simulink model "IMP_LQR_2018_Dist_Mult"  (R2018a)
settings: Solver=ode1  StartTime=0.0  StopTime=20  FixedStep=0.002  RelTol=1e-3  EnableMultiTasking=on
values from neighbouring files (symbols this model uses):
  A = [0 0 1 0 ... (first row only)    [IMP_LQR_Design_2.m]    (also in IMP_LQR_Design_C.m; IMP_LQR_Design_SepPrinc.m; IMP_LQR_Design_Seperation.m; IMP_LQR_Design_Seperation_Compare.m)
  A_aug = [A B*Cref; zeros(4,4) Aref]    [IMP_LQR_Design_2.m]    (also in IMP_LQR_Design_C.m; IMP_LQR_Design_SepPrinc.m; IMP_LQR_Design_Seperation.m; IMP_LQR_Design_Seperation_Compare.m)
  B = [0 0; 0 0; Kpp/Jp Kpy/Jp; Kyp/Jy Kyy/Jy]    [IMP_LQR_Design_2.m]    (also in IMP_LQR_Design_C.m; IMP_LQR_Design_SepPrinc.m; IMP_LQR_Design_Seperation.m; IMP_LQR_Design_Seperation_Compare.m)
  B_aug = [B; zeros(4,2)]    [IMP_LQR_Design_2.m]    (also in IMP_LQR_Design_C.m; IMP_LQR_Design_SepPrinc.m; IMP_LQR_Design_Seperation.m; IMP_LQR_Design_Seperation_Compare.m)
  C = [1 0 0 0; 0 1 0 0]    [IMP_LQR_Design_2.m]    (also in IMP_LQR_Design_C.m; IMP_LQR_Design_SepPrinc.m = [0 0 1 0; 0 1 0 0]; IMP_LQR_Design_Seperation.m; IMP_LQR_Design_Seperation_Compare.m = [0 1 0 0; 0 1 0 0])
  C_aug = [C zeros(2,4)]    [IMP_LQR_Design_2.m]    (also in IMP_LQR_Design_C.m; IMP_LQR_Design_SepPrinc.m; IMP_LQR_Design_Seperation.m; IMP_LQR_Design_Seperation_Compare.m)
  J = [J;J]    [IMP_LQR_Design_2.m]    (also in IMP_LQR_Design_C.m; IMP_LQR_Design_Seperation.m = J'; IMP_LQR_Design_Seperation_Compare.m = J'; design_C.m = place(A',C', polesj)')
  K = [K Cref]    [IMP_LQR_Design_2.m]    (also in IMP_LQR_Design_C.m; IMP_LQR_Design_SepPrinc.m; IMP_LQR_Design_Seperation.m; IMP_LQR_Design_Seperation_Compare.m)
  N = K(1:2,1:2)    [IMP_LQR_Design_2.m]    (also in IMP_LQR_Design_C.m; IMP_LQR_Design_SepPrinc.m; IMP_LQR_Design_Seperation.m; IMP_LQR_Design_Seperation_Compare.m)
  wo = 30    [IMP_LQR_Design_Seperation.m]    (also in IMP_LQR_Design_Seperation_Compare.m)
libraries: simulink x4, simulink_extras x4, dspsrcs4 x1
settings Model: ExtModeTrigDuration=5000  Creator=MLevis  LastModifiedBy=jakelangton
settings SolverCC: PositivePriorityOrder=on
settings DataIOCC: LimitDataPoints=on  SaveFormat=Array
settings OptimizationCC: LifeSpan=inf
settings DebuggingCC: SolverPrmCheckMsg=warning  SFUnexpectedBacktrackingDiag=warning  SFNoUnconditionalDefaultTransitionDiag=warning  SFExecutionAtInitializationDiag=none
settings HardwareCC: ProdBitPerPointer=32  ProdBitPerSizeT=32  ProdBitPerPtrDiffT=32  ProdLargestAtomicFloat=None  ProdIntDivRoundTo=Undefined  ProdEndianess=Unspecified  ProdWordSize=32  ProdHWDeviceType=32-bit Generic
settings ModelReferenceCC: PropagateSignalLabelsOutOfModel=off
settings RTWCC: SystemTargetFile=quarc_win64.tlc  TemplateMakefile=quarc_default_tmf  Description=QUARC Win64 Target
settings CodeAppCC: StateflowObjectComments=on
settings STFCustomTargetCC: TargetPreCompLibLocation=C:\PROGRA~3\QUARC\lib\2014a\win64\release  ConcurrentExecutionCompliant=on  GeneratePreprocessorConditionals=Disable all  SystemTargetFile=quarc_win64.tlc
settings GRTTargetCC: TargetPreCompLibLocation=C:\PROGRA~3\QUARC\lib\2014a\win64\release  TargetLangStandard=C89/C90 (ANSI)  ParMdlRefBuildCompliant=off  CompOptLevelCompliant=off  GeneratePreprocessorConditionals=Disable all  CombineOutputUpdateFcns=off  MatFileLogging=off  CPPClassGenCompliant=off  GRTInterface=on  UseToolchainInfoCompliant=off  ExtMode=on  ExtModeMexFile=quarc_comm
settings ConfigComp: CovMetricSettings=dw  CovHtmlReporting=on  CovSaveCumulativeToWorkspaceVar=on  CovSaveSingleToWorkspaceVar=on  CovExternalEMLEnable=off  CovSFcnEnable=off

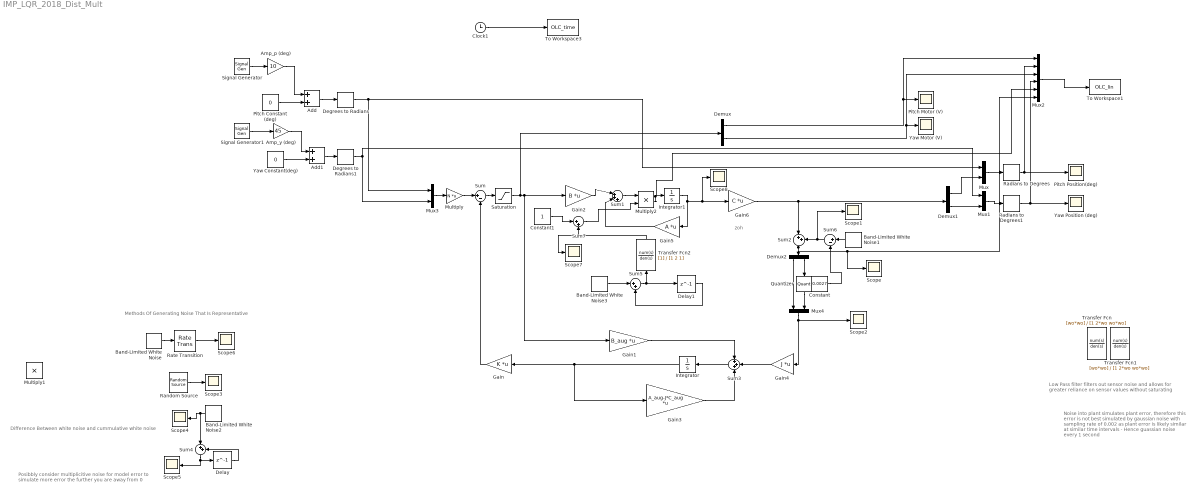
== system IMP_LQR_2018_Dist_Mult ==
  note: zoh
  note: Methods Of Generating Noise That Is Representative
  note: Noise into plant simulates plant error,
      | therefore this error is not best simulated by
      | gaussian noise with sampling rate of 0.002
      | as plant error is likely similar at similar time
      | intervals - Hence guassian noise every 1 second
  note: Low Pass filter filters out sensor noise and allows
      | for greater reliance on sensor values without saturating
  note: Difference Between white noise and cummulative white noise
  note: Posibbly consider multiplicitive noise for model error
      | to simulate more error the further you are away from 0
  Add : Sum
  Add1 : Sum
  Amp_p (deg) : Gain  Gain=10
  Amp_y (deg) : Gain  Gain=45
  Band-Limited White Noise : simulink/Sources/Band-Limited White Noise  Cov=[0.002]  Ts=0.002  seed=[23341]
  Band-Limited White Noise1 : simulink/Sources/Band-Limited White Noise  Cov=[0.0000000045 0]  Ts=0.002  seed=[23341]
  Band-Limited White Noise2 : simulink/Sources/Band-Limited White Noise  Cov=[0.00001]  Ts=.002  seed=[23341]
  Band-Limited White Noise3 : simulink/Sources/Band-Limited White Noise  Cov=[0.0000001]  Ts=.002  seed=[14252]
  Clock1 : Clock
  Constant : Constant  Value=0.0027
  Constant1 : Constant
  Degrees to Radians : simulink_extras/Transformations/Degrees to Radians
  Degrees to Radians1 : simulink_extras/Transformations/Degrees to Radians
  Delay : Delay  DelayLength=1
  Delay1 : Delay  DelayLength=1
  Demux : Demux  Outputs=2
  Demux1 : Demux  Outputs=2
  Demux2 : Demux  Outputs=2
  Gain : Gain  Gain=K  Multiplication=Matrix(K*u)
  Gain1 : Gain  Gain=B_aug  Multiplication=Matrix(K*u)
  Gain2 : Gain  Gain=B  Multiplication=Matrix(K*u)
  Gain3 : Gain  Gain=A_aug-J*C_aug  Multiplication=Matrix(K*u)
  Gain4 : Gain  Gain=J  Multiplication=Matrix(K*u)
  Gain5 : Gain  Gain=A  Multiplication=Matrix(K*u)
  Gain6 : Gain  Gain=C  Multiplication=Matrix(K*u)
  Integrator : Integrator
  Integrator1 : Integrator
  Multiply : Gain  Gain=N  Multiplication=Matrix(K*u)
  Multiply1 : Product
  Multiply2 : Product
  Mux{,1,3..4} (4 alike) : Mux  Inputs=2
  Mux2 : Mux  Inputs=6
  Pitch Constant (deg) : Constant  Value=0
  Pitch Motor (V) : Scope
  Pitch Position(deg) : Scope
  Quantizer : Quantizer  QuantizationInterval=0.03
  Radians to Degrees : simulink_extras/Transformations/Radians to Degrees
  Radians to Degrees1 : simulink_extras/Transformations/Radians to Degrees
  Random Source : dspsrcs4/Random Source  SrcType=Uniform  NormMethod=Ziggurat  CltLength=12  MinVal=0  MaxVal=1  MeanVal=0  VarVal=1  RepMode=Not repeatable  rawSeed=1  IsInherit=off  SampMode=Discrete  SampTime=1  SampFrame=1  DataType=Single  OutComplex=Real  OutputFrames=off
  Rate Transition : RateTransition  OutPortSampleTime=0.002*16
  Saturation : Saturate  UpperLimit=24  LowerLimit=-24
  Scope{,1..8} (9 alike) : Scope
  Signal Generator : SignalGenerator  Frequency=1/5
  Signal Generator1 : SignalGenerator  Frequency=1/10
  Sum : Sum  Inputs=|+-
  Sum1 : Sum  Inputs=|+++
  Sum{2,4..5,7} (4 alike) : Sum  Inputs=|++
  Sum3 : Sum  Inputs=+++
  Sum6 : Sum  Inputs=|+-
  To Workspace1 : ToWorkspace  VariableName=OLC_lin  SampleTime=-1
  To Workspace3 : ToWorkspace  VariableName=OLC_time  SampleTime=-1
  Transfer Fcn : TransferFcn  Numerator=[wo*wo]  Denominator=[1 2*wo wo*wo]
  Transfer Fcn1 : TransferFcn  Numerator=[wo*wo]  Denominator=[1 2*wo wo*wo]
  Transfer Fcn2 : TransferFcn
  Yaw Constant(deg) : Constant  Value=0
  Yaw Motor (V) : Scope
  Yaw Position (deg) : Scope
  wires:
  Degrees to Radians/1 -> Mux3/1, Mux/1
  Degrees to Radians1/1 -> Mux3/2, Mux1/1
  Signal Generator/1 -> Amp_p (deg)/1
  Pitch Constant (deg)/1 -> Add/2
  Add/1 -> Degrees to Radians/1
  Yaw Constant(deg)/1 -> Add1/2
  Amp_p (deg)/1 -> Add/1
  Signal Generator1/1 -> Amp_y (deg)/1
  Amp_y (deg)/1 -> Add1/1
  Add1/1 -> Degrees to Radians1/1
  Mux/1 -> Radians to Degrees/1
  Radians to Degrees/1 -> Mux2/2, Pitch Position(deg)/1
  Radians to Degrees1/1 -> Mux2/4, Yaw Position (deg)/1
  Demux/1 -> Mux2/1, Pitch Motor (V)/1
  Demux/2 -> Yaw Motor (V)/1, Mux2/3
  Mux1/1 -> Radians to Degrees1/1
  Mux3/1 -> Multiply/1
  Demux1/1 -> Mux/2
  Demux1/2 -> Mux1/2
  Sum/1 -> Saturation/1
  Gain1/1 -> Sum3/1
  Clock1/1 -> To Workspace3/1
  Mux2/1 -> To Workspace1/1
  Gain6/1 -> Demux1/1, Sum2/1
  Gain4/1 -> Sum3/2
  Gain3/1 -> Sum3/3
  Sum3/1 -> Integrator/1
  Integrator/1 -> Gain3/1, Gain/1
  Gain/1 -> Sum/2
  Saturation/1 -> Gain1/1, Gain2/1, Demux/1
  Multiply/1 -> Sum/1
  Integrator1/1 -> Gain5/1, Scope8/1, Gain6/1
  Gain5/1 -> Sum1/2
  Random Source/1 -> Scope3/1
  Band-Limited White Noise2/1 -> Sum4/1, Scope4/1
  Sum5/1 -> Transfer Fcn2/1, Delay1/1
  Sum4/1 -> Delay/1, Scope5/1
  Delay/1 -> Sum4/2
  Band-Limited White Noise/1 -> Rate Transition/1
  Rate Transition/1 -> Scope6/1
  Band-Limited White Noise3/1 -> Sum5/1
  Delay1/1 -> Sum5/2
  Sum2/1 -> Scope/1, Mux2/6, Demux2/1
  Sum6/1 -> Scope1/1, Sum2/2
  Band-Limited White Noise1/1 -> Sum6/1
  Constant/1 -> Sum6/2
  Mux4/1 -> Scope2/1, Gain4/1
  Demux2/1 -> Mux4/1
  Quantizer/1 -> Mux4/2
  Demux2/2 -> Quantizer/1
  Transfer Fcn2/1 -> Sum7/2, Scope7/1
  Constant1/1 -> Sum7/1
  Sum7/1 -> Multiply2/2
  Gain2/1 -> Sum1/1
  Sum1/1 -> Multiply2/1
  Multiply2/1 -> Integrator1/1, Mux2/5
